simulink model "Motion_Custom_Joint"  (R2014b)
settings: Solver=ode45  StartTime=0.0  StopTime=10.0  RelTol=1e-3
PreLoadFcn:
  | Arm_length = 0.5;
libraries: mblibv1 x9
Description:
  | Copyright 2012 The MathWorks, Inc.
settings Model: Creator=smiller  LastModifiedBy=smiller
settings DataIOCC: SignalLoggingSaveFormat=ModelDataLogs
settings OptimizationCC: ExpressionDepthLimit=2147483647  InitFltsAndDblsToZero=on
settings DebuggingCC: SaveWithParameterizedLinksMsg=none  UnderspecifiedInitializationDetection=Classic  MergeDetectMultiDrivingBlocksExec=none  FcnCallInpInsideContextMsg=UseLocalSettings  StateNameClashWarn=warning  StrictBusMsg=Warning
settings GRTTargetCC: TargetFcnLib=ansi_tfl_tmw.mat  CombineOutputUpdateFcns=off  GRTInterface=on
settings SimMechanicsCC: VisOnUpdateDiagram=on  VisDuringSimulation=on

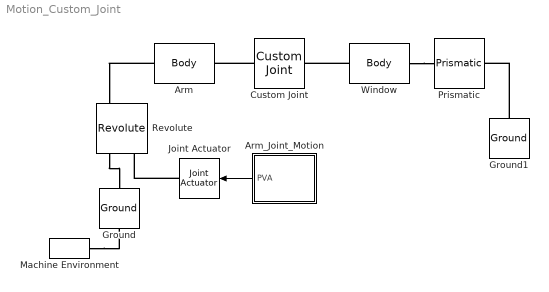
== system Motion_Custom_Joint ==
  Arm : mblibv1/Bodies/Body  LConnTagsString=CS1  RConnTagsString=CS2  UpdateFromCAD=off  DialogClass=MechanicalBodyBlock  Mass=1  MassUnits=kg  InertiaUnits=kg*m^2  Inertia=eye(3)  Shape=Cylinder  ShapeDims=[1 1]  ShapeUnits=m  ShapeUse=false  Density=1  DensityUnits=kg/m^3  DensityUse=false  GraphicsMode=MACHINE_DEFAULT  BodyColorSelMode=MACHINE_DEFAULT  BodyColor=[1 0 0]  AttachedToCS=CG  CG=Left$CG$[Arm_length/2 0 0]$CS1$CS1$m$[0 0 0]$Euler X-Y-Z$deg$WORLD$false  WorkingFrames=Left$CS1$[0 0 0]$Adjoining$Adjoining$m$[0 0 0]$Euler X-Y-Z$deg$WORLD$true#Right$CS2$[Arm_length 0 0]$CS1$CS1$m$[0 0 0]$Euler X-Y-Z$deg$WORLD$true  CGPos=[Arm_length/2 0 0]  CGRot=[0 0 0]  CS0Pos=[]  CS0Rot=[]  CS1Pos=[0 0 0]  CS1Rot=[0 0 0]  CS2Pos=[Arm_length 0 0]  CS2Rot=[0 0 0]  CS3Pos=[]  CS3Rot=[]  CS4Pos=[]  CS4Rot=[]  CS5Pos=[]  CS5Rot=[]  CS6Pos=[]  CS6Rot=[]  CS7Pos=[]  CS7Rot=[]  CS8Pos=[]  CS8Rot=[]  CS9Pos=[]  CS9Rot=[]  CS10Pos=[]  CS10Rot=[]  CS11Pos=[]  CS11Rot=[]  CS12Pos=[]  CS12Rot=[]  CS13Pos=[]  CS13Rot=[]  CS14Pos=[]  CS14Rot=[]  CS15Pos=[]  CS15Rot=[]  CS16Pos=[]  CS16Rot=[]  CS17Pos=[]  CS17Rot=[]  CS18Pos=[]  CS18Rot=[]  CS19Pos=[]  CS19Rot=[]  CS20Pos=[]  CS20Rot=[]
  Arm_Joint_Motion : Subsystem  mask{Amplitude=45, pd=20, PhaseShift=0}
      mask prompts: pd "Period (Seconds)"; PhaseShift "Phase Shift (Degrees)"
  Custom Joint : mblibv1/Joints/Custom Joint  LConnTagsString=__newl0  RConnTagsString=__newr0  UpdateFromCAD=off  NumSAPorts=0  CutJoint=off  MarkAsCut=off  Primitives=prismatic  PrimitiveProps=R1$World$[0 0 1]$revolute#P1$World$[1 0 0]$Prismatic  DialogClass=JointBlock  R1Axis=[0 0 1]  R2Axis=[]  R3Axis=[]  P1Axis=[1 0 0]  P2Axis=[]  P3Axis=[]  SAxis=[]
  Ground : mblibv1/Bodies/Ground  UpdateFromCAD=off  LeftPortType=env  RightPortType=workingframe  PhysicalDomain=Mechanical  DialogClass=GroundBlock  CoordPosition=[0 0 0]  CoordPositionUnits=m  StateVectorMgrId=-1  MachineId=[0 0]  ShowEnvPort=on  ParameterChecksum=[0 0 0 0]  TopologyChecksum=[0 0 0 0]
  Ground1 : mblibv1/Bodies/Ground  UpdateFromCAD=off  LeftPortType=env  RightPortType=workingframe  PhysicalDomain=Mechanical  DialogClass=GroundBlock  CoordPosition=[Arm_length/2 0 0]  CoordPositionUnits=m  StateVectorMgrId=-1  MachineId=[0 0]  ShowEnvPort=off  ParameterChecksum=[0 0 0 0]  TopologyChecksum=[0 0 0 0]
  Joint Actuator : mblibv1/Sensors &  Actuators/Joint Actuator  UpdateFromCAD=off  PhysicalDomain=Mechanical  PortType=blob  ActuationStyle=Motion  AngleUnits=deg  ArcVelocityUnits=deg/s  ArcAccelerationUnits=deg/s^2  CoordPositionUnits=m  VelocityUnits=m/s  AccelerationUnits=m/s^2  ForceUnits=N  TorqueUnits=N*m  ActiveIO=on  Width=3  DialogClass=MechanicalActuatorBlock  Primitive=R1  ReferenceFrame=Absolute (World)
  Machine Environment : mblibv1/Bodies/Machine Environment  Tag=Factory ground  PortType=env  PhysicalDomain=Mechanical  DialogTemplateClass=MECH.MachineEnvironment  SyncWhenCopied=off  Gravity=[0 -9.81 0]  GravityUnits=m/s^2  GravityAsSignal=off  Dimensionality=Auto-detect  AnalysisType=Forward dynamics  LinearAssemblyTolerance=1e-3  LinearAssemblyToleranceUnits=m  AngularAssemblyTolerance=1e-3  AngularAssemblyToleranceUnits=rad  ConstraintSolverType=Stabilizing  ConstraintRelTolerance=1e-4  ConstraintAbsTolerance=1e-4  UseRobustSingularityHandling=off  RedundancyAnalysisToleranceType=Automatically select tolerance  RedundancyAnalysisTolerance=1e-14  StatePerturbationType=Fixed  PerturbationSize=1e-5  VisualizeMachine=on  BodyVisualizationType=Use model default body geometries  BodyColorSelMode=Use model default  DefaultBodyColor=[1 0 0]
  Prismatic : mblibv1/Joints/Prismatic  LConnTagsString=__newl0  RConnTagsString=__newr0  UpdateFromCAD=off  NumSAPorts=0  CutJoint=off  MarkAsCut=off  Primitives=prismatic  PrimitiveProps=P1$World$[0 1 0]$prismatic  DialogClass=JointBlock  P1Axis=[0 1 0]
  Revolute : mblibv1/Joints/Revolute  LConnTagsString=__newl0|SA1  RConnTagsString=__newr0|SA1  UpdateFromCAD=off  NumSAPorts=2  CutJoint=off  MarkAsCut=off  Primitives=prismatic  PrimitiveProps=R1$World$[0 0 1]$revolute  DialogClass=JointBlock  R1Axis=[0 0 1]
  Window : mblibv1/Bodies/Body  LConnTagsString=CS1  RConnTagsString=CG  UpdateFromCAD=off  DialogClass=MechanicalBodyBlock  Mass=1  MassUnits=kg  InertiaUnits=kg*m^2  Inertia=eye(3)  Shape=Cylinder  ShapeDims=[1 1]  ShapeUnits=m  ShapeUse=false  Density=1  DensityUnits=kg/m^3  DensityUse=false  GraphicsMode=MACHINE_DEFAULT  BodyColorSelMode=MACHINE_DEFAULT  BodyColor=[1 0 0]  AttachedToCS=CG  CG=Right$CG$[-Arm_length/2 0 0]$CS1$CS1$m$[0 0 0]$Euler X-Y-Z$deg$WORLD$true  WorkingFrames=Left$CS1$[0 0 0]$Adjoining$Adjoining$m$[0 0 0]$Euler X-Y-Z$deg$WORLD$true#Right$CS2$[-Arm_length 0 0]$CS1$CS1$m$[0 0 0]$Euler X-Y-Z$deg$WORLD$false  CGPos=[-Arm_length/2 0 0]  CGRot=[0 0 0]  CS0Pos=[]  CS0Rot=[]  CS1Pos=[0 0 0]  CS1Rot=[0 0 0]  CS2Pos=[-Arm_length 0 0]  CS2Rot=[0 0 0]  CS3Pos=[]  CS3Rot=[]  CS4Pos=[]  CS4Rot=[]  CS5Pos=[]  CS5Rot=[]  CS6Pos=[]  CS6Rot=[]  CS7Pos=[]  CS7Rot=[]  CS8Pos=[]  CS8Rot=[]  CS9Pos=[]  CS9Rot=[]  CS10Pos=[]  CS10Rot=[]  CS11Pos=[]  CS11Rot=[]  CS12Pos=[]  CS12Rot=[]  CS13Pos=[]  CS13Rot=[]  CS14Pos=[]  CS14Rot=[]  CS15Pos=[]  CS15Rot=[]  CS16Pos=[]  CS16Rot=[]  CS17Pos=[]  CS17Rot=[]  CS18Pos=[]  CS18Rot=[]  CS19Pos=[]  CS19Rot=[]  CS20Pos=[]  CS20Rot=[]
  wires:
  Arm_Joint_Motion/1(PVA) -> Joint Actuator/1
  connections:
  Machine Environment/RConn1 -- Ground/LConn1
  Revolute/LConn1 -- Ground/RConn1
  Arm/LConn1 -- Revolute/RConn1
  Custom Joint/LConn1 -- Arm/RConn1
  Window/LConn1 -- Custom Joint/RConn1
  Window/RConn1 -- Prismatic/LConn1
  Ground1/RConn1 -- Prismatic/RConn1
  Joint Actuator/RConn1 -- Revolute/LConn2

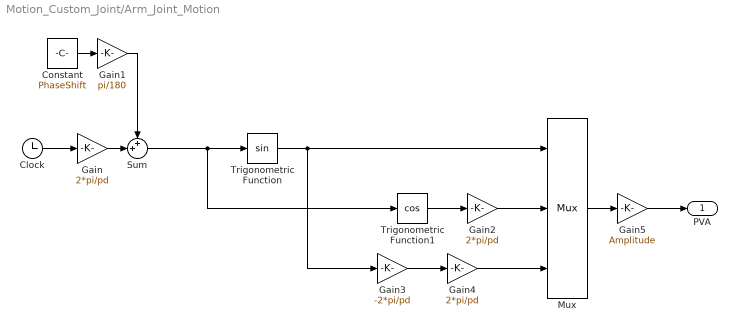
== system Motion_Custom_Joint/Arm_Joint_Motion ==
  Clock : Clock
  Constant : Constant  Value=PhaseShift
  Gain : Gain  Gain=2*pi/pd
  Gain1 : Gain  Gain=pi/180
  Gain2 : Gain  Gain=2*pi/pd
  Gain3 : Gain  Gain=-2*pi/pd
  Gain4 : Gain  Gain=2*pi/pd
  Gain5 : Gain  Gain=Amplitude
  Mux : Mux  Inputs=3
  Sum : Sum  Inputs=++|
  Trigonometric Function : Trigonometry
  Trigonometric Function1 : Trigonometry  Operator=cos
  PVA : Outport
  wires:
  Gain4/1 -> Mux/3
  Gain3/1 -> Gain4/1
  Gain2/1 -> Mux/2
  Trigonometric Function1/1 -> Gain2/1
  Gain5/1 -> PVA/1
  Mux/1 -> Gain5/1
  Trigonometric Function/1 -> Gain3/1, Mux/1
  Sum/1 -> Trigonometric Function1/1, Trigonometric Function/1
  Gain1/1 -> Sum/1
  Constant/1 -> Gain1/1
  Gain/1 -> Sum/2
  Clock/1 -> Gain/1
